simulink model "MPC4_QUES1_MPCLinear"  (R2024b)
settings: Solver=VariableStepAuto  StartTime=0.0  StopTime=30  RelTol=1e-3
libraries: mpclib x1
settings Model: Creator=Reza Shahriari  LastModifiedBy=Reza Shahriari

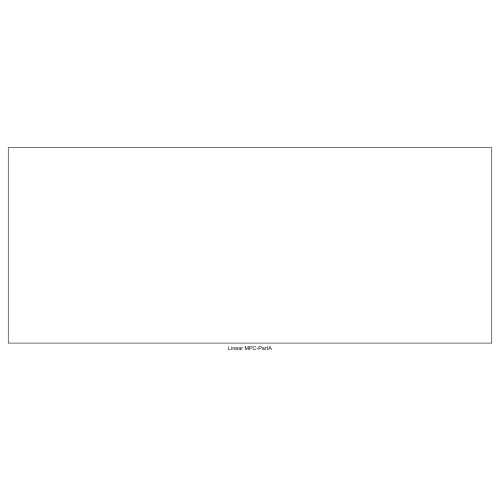
[thumbnail: Simulink's stored preview of the top-level diagram]
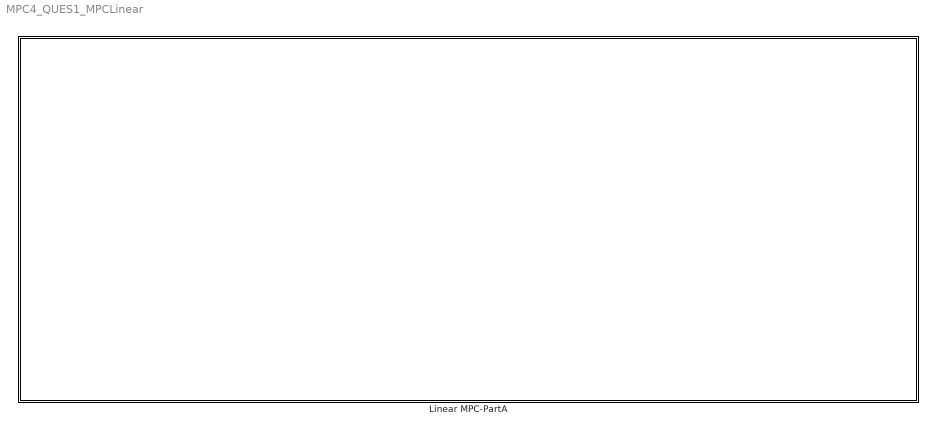
== system MPC4_QUES1_MPCLinear ==
  Linear MPC-PartA : Subsystem

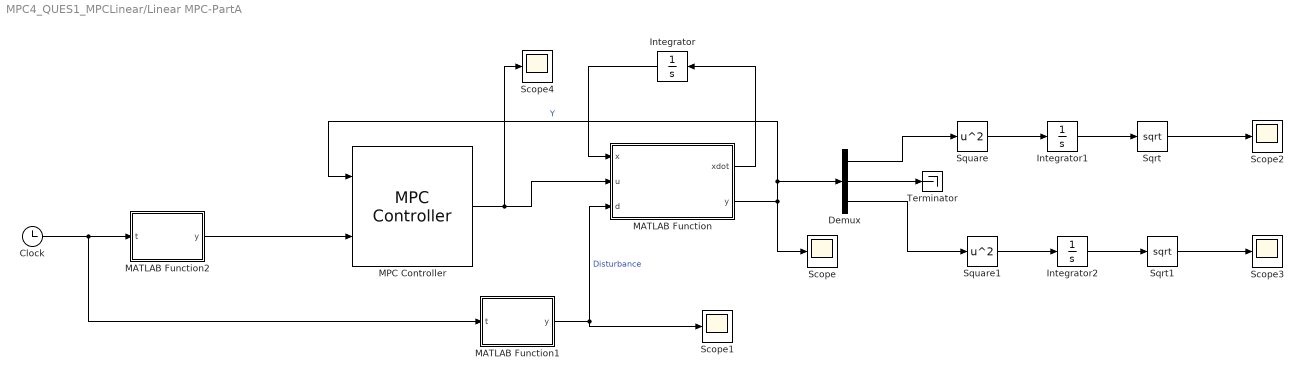
== system MPC4_QUES1_MPCLinear/Linear MPC-PartA ==
  Clock : Clock
  Demux : Demux  Outputs=3
  Integrator : Integrator  InitialCondition=[0;0;0;0]
  Integrator1 : Integrator
  Integrator2 : Integrator
  MATLAB Function : MATLAB Function  TreatAsAtomicUnit=on
  MATLAB Function1 : MATLAB Function  TreatAsAtomicUnit=on
  MATLAB Function2 : MATLAB Function  TreatAsAtomicUnit=on
  MPC Controller : mpclib/MPC Controller  SCDEnableBlockLinearizationSpecification=on  mpcobj=mpc1  is_multiple=0  enable_value=0  return_u0=off  updateMPCinCallerWorkspace=on  md_inport=off  mv_inport=off  uref_inport=off  return_cost=off  return_mvseq=off  return_qpstatus=off  return_xseq=off  return_state=off  return_ovseq=off  state_inport=off  umin_inport=off  umax_inport=off  ymin_inport=off  ymax_inport=off  cc_inport=off  ywt_inport=off  uwt_inport=off  duwt_inport=off  rhoeps_inport=off  pm_inport=off  MaximumP=10  HorizonChoice=FixedHorizon  n_ts=0.01  n_p=100  n_mv=1  n_md=0  n_ud=0  n_mo=3  n_uo=0  BlockDataType=double  SampleTimeInherited=off  switch_inport=off
  Scope{,1..4} (5 alike) : Scope
  Sqrt : Sqrt
  Sqrt1 : Sqrt
  Square : Math  Operator=square
  Square1 : Math  Operator=square
  Terminator : Terminator
  wires:
  MATLAB Function1/1(y) -> Scope1/1, MATLAB Function/3(d)  "Disturbance"
  MPC Controller/1 -> Scope4/1, MATLAB Function/2(u)
  MATLAB Function/1(xdot) -> Integrator/1
  MATLAB Function/2(y) -> Demux/1, MPC Controller/1, Scope/1  "Y"
  Integrator/1 -> MATLAB Function/1(x)
  MATLAB Function2/1(y) -> MPC Controller/2
  Clock/1 -> MATLAB Function1/1(t), MATLAB Function2/1(t)
  Square/1 -> Integrator1/1
  Integrator1/1 -> Sqrt/1
  Integrator2/1 -> Sqrt1/1
  Square1/1 -> Integrator2/1
  Demux/1 -> Square/1
  Demux/3 -> Square1/1
  Demux/2 -> Terminator/1
  Sqrt/1 -> Scope2/1
  Sqrt1/1 -> Scope3/1

== matlab function MPC4_QUES1_MPCLinear/Linear MPC-PartA/MATLAB Function1 ==
  data: t input; y output
function y = Disturbance(t)

if t>=4 & t<5 
    y = t-4;
elseif t>=5 & t<7
    y = 1;
elseif t>=7 & t<8
    y = -t+8;
else 
    y = 0;
end

== matlab function MPC4_QUES1_MPCLinear/Linear MPC-PartA/MATLAB Function ==
  data: x input; xdot output; u input; y output; d input
function [xdot,y]= SystemDynamics(x,u,d)

% Parameter Definition
Ms = 2500;
Mu = 320;
ks = 80000;
ku = 500000;
cs = 350;
cu = 15020;

A = [0 1 0 0;
     0 -cs/Ms -ks/Ms cs/Ms;
     0 1 0 -1;
     -ku/Mu cs/Mu (ks+ku)/Mu -(cs+cu)/Mu];
     
B = [0; 1/Ms; 0; -1/Mu];  % Input matrix

C = [1 0 0 0; 0 1 0 0; 0 0 1 0];

Ad = [0.9241    0.0945   -0.0672    0.0013;
   -2.0392    0.8450   -0.6570    0.0178;
    0.8830    0.0843   -0.1675    0.0021;
    1.2927    0.1390   -1.8258   -0.0591];

Bd = [    0.1053;
    2.2534;
   -0.8123;
  -51.0695];

Cd = C;


Diss = [0; cs*cu/(Ms*Mu); -cu/Mu; (cu/Mu)*(ku*cu-cs*Mu-cu*Mu)];

xdot = A*x + B*u + Diss*d;
y = C*x;

== matlab function MPC4_QUES1_MPCLinear/Linear MPC-PartA/MATLAB Function2 ==
  data: y output; t input
function y = fcn(t)

y = [0;0;0];
